simulink model "observabilidades_prev_versions"  (R2024a)
settings: Solver=VariableStepAuto  StartTime=0.0  StopTime=30  RelTol=1e-3
values from neighbouring files (symbols this model uses):
  A = [0 1 0 0 ... (first row only)    [code_cte_small.m]    (also in lab1.m)
  Afcc = inv(T) * A * T    [code_cte_small.m]    (also in lab1.m)
  Afco = inv(Q)*A*Q    [code_cte_small.m]    (also in lab1.m)
  B = [0 ... (first row only)    [code_cte_small.m]    (also in lab1.m)
  Bfcc = inv(T) * B    [code_cte_small.m]    (also in lab1.m)
  Bfco = inv(Q) * B    [code_cte_small.m]    (also in lab1.m)
  C = [1 0 0 0]    [code_cte_small.m]    (also in lab1.m)
  Cfcc = C * T    [code_cte_small.m]    (also in lab1.m)
  Cfco = C * Q    [code_cte_small.m]    (also in lab1.m)
  E = [0 ... (first row only)    [code_cte_small.m]    (also in lab1.m)
  Efcc = inv(T)*E    [code_cte_small.m]    (also in lab1.m)
  Efco = inv(Q) * E    [code_cte_small.m]    (also in lab1.m)
  k_obs_F_matriz = inv(matriz_P_f)*k_cachuchita_f'    [code_cte_small.m]    (also in lab1.m)
  k_obs_FCC_matriz = inv(matriz_P)*k_cachuchita'    [code_cte_small.m]    (also in lab1.m)
  k_obs_FCO_matriz = inv(matriz_P_fco)*k_cachuchita_fco'    [code_cte_small.m]    (also in lab1.m)
settings Model: Creator=Usuario  LastModifiedBy=Usuario

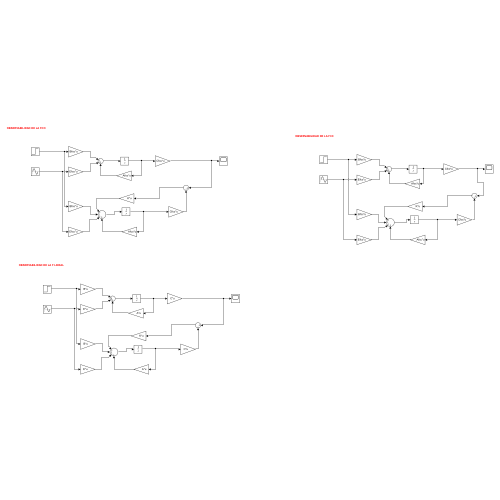
[thumbnail: Simulink's stored preview of the top-level diagram]
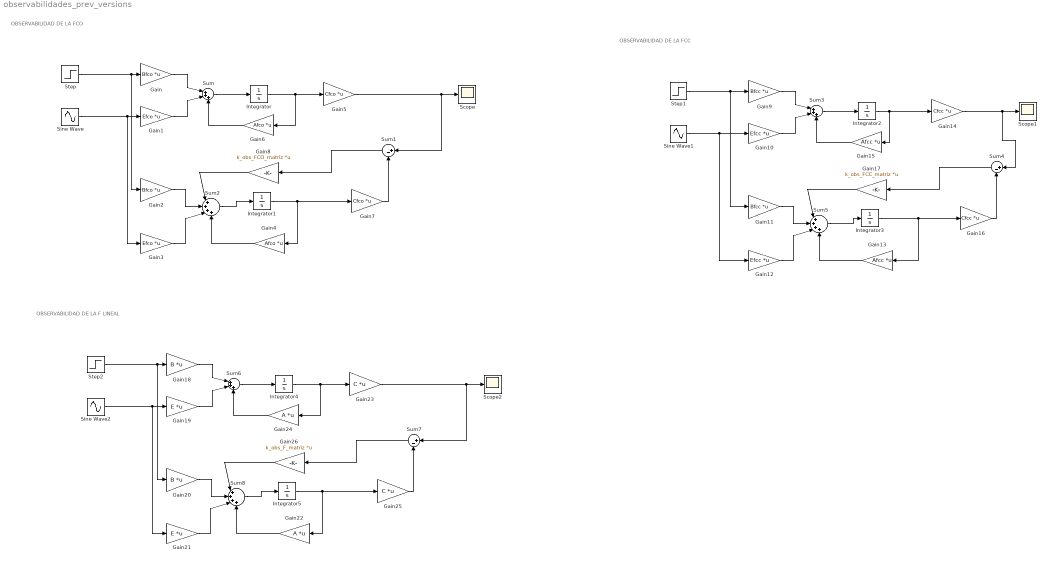
== system observabilidades_prev_versions ==
  note: OBSERVABILIDAD DE LA FCO
  note: OBSERVABILIDAD DE LA FCC
  note: OBSERVABILIDAD DE LA F LINEAL
  Gain : Gain  Gain=Bfco  Multiplication=Matrix(K*u)
  Gain1 : Gain  Gain=Efco  Multiplication=Matrix(K*u)
  Gain10 : Gain  Gain=Efcc  Multiplication=Matrix(K*u)
  Gain11 : Gain  Gain=Bfcc  Multiplication=Matrix(K*u)
  Gain12 : Gain  Gain=Efcc  Multiplication=Matrix(K*u)
  Gain13 : Gain  Gain=Afcc  Multiplication=Matrix(K*u)
  Gain14 : Gain  Gain=Cfcc  Multiplication=Matrix(K*u)
  Gain15 : Gain  Gain=Afcc  Multiplication=Matrix(K*u)
  Gain16 : Gain  Gain=Cfcc  Multiplication=Matrix(K*u)
  Gain17 : Gain  Gain=k_obs_FCC_matriz  Multiplication=Matrix(K*u)
  Gain18 : Gain  Gain=B  Multiplication=Matrix(K*u)
  Gain19 : Gain  Gain=E  Multiplication=Matrix(K*u)
  Gain2 : Gain  Gain=Bfco  Multiplication=Matrix(K*u)
  Gain20 : Gain  Gain=B  Multiplication=Matrix(K*u)
  Gain21 : Gain  Gain=E  Multiplication=Matrix(K*u)
  Gain22 : Gain  Gain=A  Multiplication=Matrix(K*u)
  Gain23 : Gain  Gain=C  Multiplication=Matrix(K*u)
  Gain24 : Gain  Gain=A  Multiplication=Matrix(K*u)
  Gain25 : Gain  Gain=C  Multiplication=Matrix(K*u)
  Gain26 : Gain  Gain=k_obs_F_matriz  Multiplication=Matrix(K*u)
  Gain3 : Gain  Gain=Efco  Multiplication=Matrix(K*u)
  Gain4 : Gain  Gain=Afco  Multiplication=Matrix(K*u)
  Gain5 : Gain  Gain=Cfco  Multiplication=Matrix(K*u)
  Gain6 : Gain  Gain=Afco  Multiplication=Matrix(K*u)
  Gain7 : Gain  Gain=Cfco  Multiplication=Matrix(K*u)
  Gain8 : Gain  Gain=k_obs_FCO_matriz  Multiplication=Matrix(K*u)
  Gain9 : Gain  Gain=Bfcc  Multiplication=Matrix(K*u)
  Integrator{,1..5} (6 alike) : Integrator
  Scope : Scope
  Scope1 : Scope
  Scope2 : Scope
  Sine Wave : Sin  Frequency=5  SampleTime=0
  Sine Wave1 : Sin  Frequency=5  SampleTime=0
  Sine Wave2 : Sin  Frequency=5  SampleTime=0
  Step : Step  SampleTime=0
  Step1 : Step  SampleTime=0
  Step2 : Step  SampleTime=0
  Sum : Sum  Inputs=|+++
  Sum1 : Sum  Inputs=|+-
  Sum2 : Sum  Inputs=|++++
  Sum3 : Sum  Inputs=|+++
  Sum4 : Sum  Inputs=|+-
  Sum5 : Sum  Inputs=|++++
  Sum6 : Sum  Inputs=|+++
  Sum7 : Sum  Inputs=|+-
  Sum8 : Sum  Inputs=|++++
  wires:
  Sine Wave/1 -> Gain3/1, Gain1/1
  Step/1 -> Gain2/1, Gain/1
  Gain/1 -> Sum/1
  Gain1/1 -> Sum/2
  Gain6/1 -> Sum/3
  Sum/1 -> Integrator/1
  Integrator/1 -> Gain5/1, Gain6/1
  Gain5/1 -> Sum1/1, Scope/1
  Gain7/1 -> Sum1/2
  Sum1/1 -> Gain8/1
  Sum2/1 -> Integrator1/1
  Integrator1/1 -> Gain4/1, Gain7/1
  Gain8/1 -> Sum2/1
  Gain2/1 -> Sum2/2
  Gain3/1 -> Sum2/3
  Gain4/1 -> Sum2/4
  Gain14/1 -> Sum4/1, Scope1/1
  Gain13/1 -> Sum5/4
  Integrator2/1 -> Gain14/1, Gain15/1
  Sum3/1 -> Integrator2/1
  Gain11/1 -> Sum5/2
  Integrator3/1 -> Gain13/1, Gain16/1
  Gain16/1 -> Sum4/2
  Gain15/1 -> Sum3/3
  Sum5/1 -> Integrator3/1
  Gain10/1 -> Sum3/2
  Gain12/1 -> Sum5/3
  Gain17/1 -> Sum5/1
  Gain9/1 -> Sum3/1
  Sine Wave1/1 -> Gain12/1, Gain10/1
  Sum4/1 -> Gain17/1
  Step1/1 -> Gain11/1, Gain9/1
  Gain23/1 -> Sum7/1, Scope2/1
  Gain22/1 -> Sum8/4
  Integrator4/1 -> Gain23/1, Gain24/1
  Sum6/1 -> Integrator4/1
  Gain20/1 -> Sum8/2
  Integrator5/1 -> Gain22/1, Gain25/1
  Gain25/1 -> Sum7/2
  Gain24/1 -> Sum6/3
  Sum8/1 -> Integrator5/1
  Gain19/1 -> Sum6/2
  Gain21/1 -> Sum8/3
  Gain26/1 -> Sum8/1
  Gain18/1 -> Sum6/1
  Sine Wave2/1 -> Gain21/1, Gain19/1
  Sum7/1 -> Gain26/1
  Step2/1 -> Gain20/1, Gain18/1
